simulink model "BikeModelDynWheels"  (R2017b)
settings: Solver=VariableStepAuto  StartTime=0.0  StopTime=10.0  RelTol=1e-3
undefined symbols (not defined in the file): b_contact, C_F_alpha, C_F_kappa, Cylinder, Dphi0, Dpsi0, epsilon, g, k_contact, lengthFF, lengthRF, lengthRW, locY, locZ, massRW, mB, mH, Parts_Lib, radiusRW, sigma, X, xPla, Y, yPla, Z, zPla
libraries: sm_lib x24, nesl_utility x18, vrlib x8, dspsrcs4 x1
(part 2 of 2)

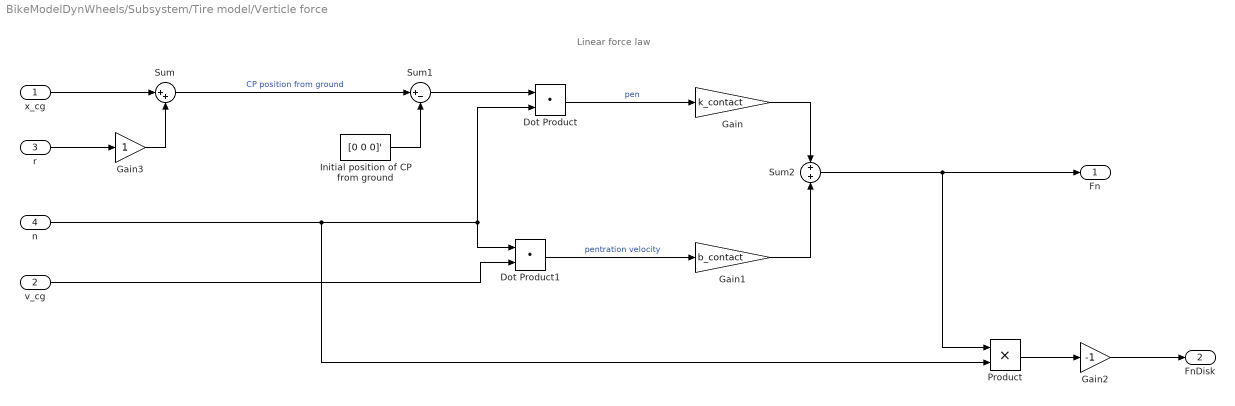
== system BikeModelDynWheels/Subsystem/Tire model/Verticle force ==
  note: Linear force law
  x_cg : Inport
  v_cg : Inport  Port=2
  r : Inport  Port=3
  n : Inport  Port=4
  Dot Product : DotProduct  InputSameDT=on  OutDataTypeStr=Inherit: Inherit via internal rule
  Dot Product1 : DotProduct  InputSameDT=on  OutDataTypeStr=Inherit: Inherit via internal rule
  Gain : Gain  Gain=k_contact
  Gain1 : Gain  Gain=b_contact
  Gain2 : Gain  Gain=-1
  Gain3 : Gain
  Initial position of CP from ground : Constant  Value=[0 0 0]'
  Product : Product
  Sum : Sum  Inputs=|++
  Sum1 : Sum  Inputs=|+-
  Sum2 : Sum
  Fn : Outport
  FnDisk : Outport  Port=2
  wires:
  x_cg/1 -> Sum/1
  Sum/1 -> Sum1/1  "CP position from ground"
  Initial position of CP from ground/1 -> Sum1/2
  Sum1/1 -> Dot Product/1
  Dot Product/1 -> Gain/1  "pen"
  v_cg/1 -> Dot Product1/2
  Dot Product1/1 -> Gain1/1  "pentration velocity"
  Gain1/1 -> Sum2/2
  Sum2/1 -> Product/1, Fn/1
  Product/1 -> Gain2/1
  n/1 -> Product/2, Dot Product1/1, Dot Product/2
  Gain/1 -> Sum2/1
  r/1 -> Gain3/1
  Gain3/1 -> Sum/2
  Gain2/1 -> FnDisk/1

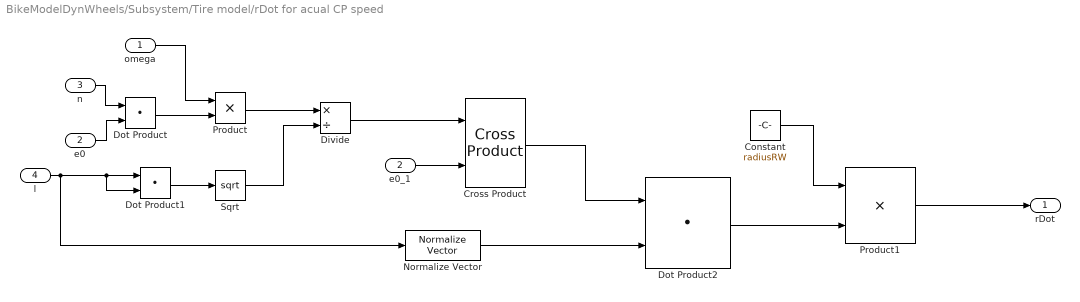
== system BikeModelDynWheels/Subsystem/Tire model/rDot for acual CP speed ==
  omega : Inport
  e0 : Inport  Port=2
  n : Inport  Port=3
  l : Inport  Port=4
  Constant : Constant  Value=radiusRW
  Cross Product : vrlib/Utilities/Cross Product
      settings: SourceProductBaseCode=VR
  Divide : Product  Inputs=*/
  Dot Product : DotProduct  InputSameDT=on  OutDataTypeStr=Inherit: Inherit via internal rule
  Dot Product1 : DotProduct  InputSameDT=on  OutDataTypeStr=Inherit: Inherit via internal rule
  Dot Product2 : DotProduct  InputSameDT=on  OutDataTypeStr=Inherit: Inherit via internal rule
  Normalize Vector : vrlib/Utilities/Normalize Vector  maxzero=0
      settings: SourceProductName=Simulink 3D Animation  SourceProductBaseCode=VR
  Product : Product
  Product1 : Product
  Sqrt : Sqrt  SaturateOnIntegerOverflow=on
  e0_1 : InportShadow  Port=2
  rDot : Outport
  wires:
  n/1 -> Dot Product/1
  e0/1 -> Dot Product/2
  Dot Product/1 -> Product/2
  omega/1 -> Product/1
  Product/1 -> Divide/1
  l/1 -> Normalize Vector/1, Dot Product1/2, Dot Product1/1
  Dot Product1/1 -> Sqrt/1
  Sqrt/1 -> Divide/2
  Divide/1 -> Cross Product/1
  e0_1/1 -> Cross Product/2
  Cross Product/1 -> Dot Product2/1
  Dot Product2/1 -> Product1/2
  Product1/1 -> rDot/1
  Normalize Vector/1 -> Dot Product2/2
  Constant/1 -> Product1/1
